simulink model "VCMGCM1962020b_v2"  (R2020b)
settings: Solver=FixedStepDiscrete  StartTime=0.0  StopTime=10.0  FixedStep=0.005  RelTol=1e-3  EnableMultiTasking=on
PreLoadFcn:
  | try, model_open; catch, disp('Error occurred while executing model pre-load callback: model_open.m'); disp('Please assure that the MATLAB working directory is set to the model directory before opening.'); end
InitFcn:
  | try, model_open; catch, end
undefined symbols (not defined in the file): Bridge, GCM, H, raptor_get_param_eval, raptor_get_safe_string, raptor_xcp_function
libraries: Blocks_lib x1165, Raptor_lib x665, simulink x62, VCM_lib x5
(part 7 of 23)

== system VCMGCM1962020b_v2/Fgnd/Virtual Sensors/Driver Inputs/Brk ==
  note: TBC
  Data : Inport
  BrkPos : Subsystem
  Bus Selector1 : BusSelector  OutputSignals=Sensors.Sensors.Driver.BrkSwInpt.BrkSwInptVld [Bool],Sensors.Sensors.Driver.BrkSwInpt.BrkSwInpt [Bool]
  Header : Blocks_lib/Header  width=Portrait  addtext=''
  Meas&Ovrd : Blocks_lib/Meas&Ovrd  nam='BrkSw'  name_source=Parameter  view_as=Number  enum_struct={}  gain=1  min=-inf  max=inf  precision=''  units='Bool'  help='Brake Switch position'  group='Virtual Sensors | Driver Input'
  Multiport Switch : MultiPortSwitch  DataPortOrder=Zero-based contiguous  Inputs=2  zeroidx=on
  Relational Operator : RelationalOperator  OutDataTypeStr=boolean  RndMeth=Simplest
  Zero-Order Hold : ZeroOrderHold  SampleTime=-1
  raptor_adjustment : Raptor_lib/Data Storage/raptor_adjustment  paramName='BrkSwSource'  nameSource=Parameter  initValue=0  dataType=double  storage=Calibration  calDispType=Number  calEnum={}  calGain=1.0  calOffset=0.0  calMax=inf  calMin=-inf  calFormat='-1'  calUnit='Bool'  calHelp=' 0 = simple switch., 1 = dual sensor switch'  calAccess=1  calFunction='Virtual Sensors | Driver Input'  calDispHeaders=off  calColHeaders={'Col1' 'Col2' 'Col3'}  calRowHeaders={'Row1' 'Row2' 'Row3'}
      settings: SourceProductName=Raptor
  raptor_adjustment1 : Raptor_lib/Data Storage/raptor_adjustment  paramName='BrkPos_Swtch_Thr'  nameSource=Parameter  initValue=20  dataType=double  storage=Calibration  calDispType=Number  calEnum={}  calGain=1.0  calOffset=0.0  calMax=inf  calMin=-inf  calFormat='-1'  calUnit='%'  calHelp=' Value of Pos Sensor to set Vitual brk switch to on'  calAccess=1  calFunction='Virtual Sensors | Driver Input'  calDispHeaders=off  calColHeaders={'Col1' 'Col2' 'Col3'}  calRowHeaders={'Row1' 'Row2' 'Row3'}
      settings: SourceProductName=Raptor
  Vld : Outport  VectorParamsAs1DForOutWhenUnconnected=off
  Brk : Outport  Port=2  VectorParamsAs1DForOutWhenUnconnected=off
  Pos : Outport  Port=3  VectorParamsAs1DForOutWhenUnconnected=off
  PosVld : Outport  Port=4  VectorParamsAs1DForOutWhenUnconnected=off
  wires:
  Data/1 -> BrkPos/1(Data), Bus Selector1/1
  Meas&Ovrd/1 -> Multiport Switch/2
  Bus Selector1/1 -> Zero-Order Hold/1  "<BrkSwInptVld [Bool]>"
  Bus Selector1/2 -> Meas&Ovrd/1  "<BrkSwInpt [Bool]>"
  Zero-Order Hold/1 -> Vld/1  "BrkSwVld [Bool]"
  BrkPos/1(Vld) -> PosVld/1
  BrkPos/2(%) -> Relational Operator/1, Pos/1
  raptor_adjustment1/1 -> Relational Operator/2
  raptor_adjustment/1 -> Multiport Switch/1
  Relational Operator/1 -> Multiport Switch/3
  Multiport Switch/1 -> Brk/1

== system VCMGCM1962020b_v2/Fgnd/Virtual Sensors/Driver Inputs/ParkBrake ==
  Data : Inport
  Bus Selector : BusSelector  OutputSignals=Sensors.CAN.Other.BCM.CCVS1_BCM.Parking_Brak_Switch.Parking_Brak_SwitchVld [Bool],Sensors.CAN.Other.BCM.CCVS1_BCM.Parking_Brak_Switch.Parking_Brak_Switch [enum]
  Constant : Constant
  Constant1 : Constant  Value=boolean(0)
  Constant2 : Constant  Value=boolean(1)
  Equal : RelationalOperator  Operator===  OutDataTypeStr=boolean  RndMeth=Simplest
  Header : Blocks_lib/Header  width=Portrait  addtext=''
  Multiport Switch : MultiPortSwitch  DataPortOrder=Zero-based contiguous  Inputs=2  zeroidx=on
  Multiport Switch1 : MultiPortSwitch  DataPortOrder=Zero-based contiguous  Inputs=2  zeroidx=on
  raptor_adjustment : Raptor_lib/Data Storage/raptor_adjustment  paramName='PrkBrk_Dflt'  nameSource=Parameter  initValue=0.00  dataType=boolean  storage=Calibration  calDispType=Number  calEnum={'False', 'True'}  calGain=1.0  calOffset=0.0  calMax=inf  calMin=-inf  calFormat='-1'  calUnit=''  calHelp=''  calAccess=1  calFunction=raptor_xcp_function(gcb)  calDispHeaders=off  calColHeaders={'Col1' 'Col2' 'Col3'}  calRowHeaders={'Row1' 'Row2' 'Row3'}
      settings: SourceProductName=Raptor
  raptor_measurement : Raptor_lib/Data Storage/raptor_measurement  paramName='PrkBrk'  nameSource=Parameter  calDispType=Number  calEnum={'False', 'True'}  calGain=1.0  calOffset=0.0  calMax=inf  calMin=-inf  calFormat='-1'  calUnit=''  calHelp=''  calAccess=1  calFunction=raptor_xcp_function(gcb)  calVisible=on
      settings: SourceProductName=Raptor
  Prk : Outport
  wires:
  Data/1 -> Bus Selector/1
  Bus Selector/2 -> Equal/1  "<Parking_Brak_Switch [enum]>"
  Constant/1 -> Equal/2
  Bus Selector/1 -> Multiport Switch/1  "<Parking_Brak_SwitchVld [Bool]>"
  Multiport Switch/1 -> Prk/1, raptor_measurement/1  "Prk [Bool]"
  Equal/1 -> Multiport Switch1/1
  Constant1/1 -> Multiport Switch1/2
  Constant2/1 -> Multiport Switch1/3
  Multiport Switch1/1 -> Multiport Switch/3
  raptor_adjustment/1 -> Multiport Switch/2

== system VCMGCM1962020b_v2/Fgnd/Virtual Sensors/Driver Inputs/VehPwrMode ==
  Data : Inport
  Bus Selector : BusSelector  OutputSignals=Sensors.Sensors.Volt.Wake [Bool]
  EnumCnst : Blocks_lib/EnumCnst  val='Off'  typ=uint8  enum=EnumLst.VehPwrMode
  EnumCnst1 : Blocks_lib/EnumCnst  val='Run'  typ=uint8  enum=EnumLst.VehPwrMode
  Header : Blocks_lib/Header  width=Portrait  addtext=''
  Multiport Switch : MultiPortSwitch  DataPortOrder=Zero-based contiguous  Inputs=2  zeroidx=on
  enum : Outport  VectorParamsAs1DForOutWhenUnconnected=off
  wires:
  Multiport Switch/1 -> enum/1
  Data/1 -> Bus Selector/1
  Bus Selector/1 -> Multiport Switch/1  "<Wake [Bool]>"
  EnumCnst/1 -> Multiport Switch/2
  EnumCnst1/1 -> Multiport Switch/3

== system VCMGCM1962020b_v2/Fgnd/Virtual Sensors/PDU/HVAccCur ==
  note: Note: This value is used downstream to calculate inverter and charger current limits.
      | Therefore, neither inverter nor charger current should be included in this calculation.
  Data : Inport
  Bus Selector : BusSelector  OutputSignals=VirtualSensors.DCDC.DCDCInptCur [A]
  Header : Blocks_lib/Header  width=Portrait  addtext=''
  raptor_measurement : Raptor_lib/Data Storage/raptor_measurement  paramName='HVAccCur'  nameSource=Parameter  calDispType=Number  calEnum={'Disabled', 'Enabled'}  calGain=1  calOffset=0  calMax=inf  calMin=-inf  calFormat=''  calUnit='A'  calHelp='High-voltage accessory current'  calAccess=1  calFunction='Virtual Sensors | PDU'  calVisible=on
      settings: SourceProductName=Raptor
  A : Outport  VectorParamsAs1DForOutWhenUnconnected=off
  wires:
  Data/1 -> Bus Selector/1
  Bus Selector/1 -> raptor_measurement/1, A/1  "<DCDCInptCur [A]>"

== system VCMGCM1962020b_v2/Fgnd/Virtual Sensors/PDU/HVBusIso ==
  Data : Inport
  Bus Selector : BusSelector  OutputSignals=Sensors.CAN.Batt.HVES1_Status1.PSV_ISO_TEST_State.PSV_ISO_TEST_StateVld [Bool],Sensors.CAN.Batt.HVES1_Status1.PSV_ISO_TEST_State.PSV_ISO_TEST_State []
  Compare To Constant : simulink/Logic and Bit Operations/Compare To Constant  relop=>=  const=4  OutDataTypeStr=boolean
  Compare To Constant1 : simulink/Logic and Bit Operations/Compare To Constant  relop=<=  const=5  OutDataTypeStr=boolean
  Header : Blocks_lib/Header  width=Portrait  addtext=''
  OR : Logic  Operator=OR  AllPortsSameDT=off  OutDataTypeStr=boolean
  Zero-Order Hold : ZeroOrderHold  SampleTime=-1
  Zero-Order Hold1 : ZeroOrderHold  SampleTime=-1
  Vld : Outport  VectorParamsAs1DForOutWhenUnconnected=off
  "ISOTst " : Outport  Port=2  VectorParamsAs1DForOutWhenUnconnected=off
  ISOFailed : Outport  Port=3  VectorParamsAs1DForOutWhenUnconnected=off
  wires:
  Data/1 -> Bus Selector/1
  Bus Selector/2 -> Compare To Constant1/1, Compare To Constant/1, Zero-Order Hold1/1  "<PSV_ISO_TEST_State []>"
  Bus Selector/1 -> Zero-Order Hold/1  "<PSV_ISO_TEST_StateVld [Bool]>"
  Zero-Order Hold/1 -> Vld/1
  Zero-Order Hold1/1 -> "ISOTst "/1  "PSV_ISO_Test_State [uint8]"
  Compare To Constant/1 -> OR/1
  Compare To Constant1/1 -> OR/2
  OR/1 -> ISOFailed/1

== system VCMGCM1962020b_v2/Fgnd/Virtual Sensors/PDU/HVBusVolt ==
  note: TBC
  Data : Inport
  Bus Selector : BusSelector  OutputSignals=Sensors.CAN.DrvInvtr.EM3.EM3DCv.EM3_InverterDcV.EM3_InverterDcVVld [Bool],Sensors.CAN.DrvInvtr.EM3.EM3DCv.EM3_InverterDcV.EM3_InverterDcV [V]
  HV Bus Voltage : Subsystem  Commented=on  mask{nam='HVBusVolt', group='Virtual Sensors | PDU'}
      mask prompts: nam "Name"
      mask Display: disp(['High-Voltage Bus Voltage\n' nam]);
  Header : Blocks_lib/Header  width=Portrait  addtext=''
  Vld : Outport  VectorParamsAs1DForOutWhenUnconnected=off
  V : Outport  Port=2  VectorParamsAs1DForOutWhenUnconnected=off
  wires:
  Data/1 -> Bus Selector/1, HV Bus Voltage/1(Data)
  Bus Selector/1 -> Vld/1  "<EM3_InverterDcVVld [Bool]>"
  Bus Selector/2 -> V/1  "<EM3_InverterDcV [V]>"

== system VCMGCM1962020b_v2/Fgnd/Virtual Sensors/PDU/MainCntrClosed ==
  Data : Inport
  Bus Selector : BusSelector  OutputSignals=VirtualSensors.PDU.MainPosCntrClosedVld [Bool],VirtualSensors.PDU.MainNegCntrClosedVld [Bool],VirtualSensors.PDU.MainPosCntrClosed [Bool],VirtualSensors.PDU.MainNegCntrClosed [Bool]
  Header : Blocks_lib/Header  width=Portrait  addtext=''
  Logical Operator : Logic  OutDataTypeStr=boolean
  Logical Operator1 : Logic  OutDataTypeStr=boolean
  Vld : Outport  VectorParamsAs1DForOutWhenUnconnected=off
  Bool : Outport  Port=2  VectorParamsAs1DForOutWhenUnconnected=off
  wires:
  Data/1 -> Bus Selector/1
  Bus Selector/1 -> Logical Operator/1  "<MainPosCntrClosedVld [Bool]>"
  Logical Operator/1 -> Vld/1
  Bus Selector/2 -> Logical Operator/2  "<MainNegCntrClosedVld [Bool]>"
  Bus Selector/3 -> Logical Operator1/1  "<MainPosCntrClosed [Bool]>"
  Bus Selector/4 -> Logical Operator1/2  "<MainNegCntrClosed [Bool]>"
  Logical Operator1/1 -> Bool/1

== system VCMGCM1962020b_v2/Fgnd/Virtual Sensors/Vehicle/Range ==
  Odom : Inport
  Data : Inport  Port=2
  Bus Selector : BusSelector  OutputSignals=VirtualSensors.Batt.BattSOC [%]
  CntrLoop : Subsystem  TreatAsAtomicUnit=on  mask(CntrLoop){init=0, typ=uint16, rstval=2000}
      mask prompts: init "Initial Value"; typ "Data Type"; rstval "Reset at:"
      mask init:
      | cb = gcb;
      | 
      | % --- Parameter Setting
      | set_param([cb '/Constant'], 'OutDataTypeStr', typ);
      mask TypeOptions typ: double | single | int8 | uint8 | int16 | uint16 | int32 | uint32 | boolean
      mask Display: disp(['Loop Counter\nReset at ' num2str(rstval)]);
  Compare To Constant : simulink/Logic and Bit Operations/Compare To Constant  relop===  const=0  OutDataTypeStr=boolean
  Filt : Blocks_lib/Filt  nam='RangeEstFiltTC'  group='Virtual Sensors | Speed'  samptime=samptime
  Header : Blocks_lib/Header  width=Portrait  addtext=''
  Product : Product
  RangeGain : Subsystem
  Subsystem1 : Subsystem
  raptor_measurement : Raptor_lib/Data Storage/raptor_measurement  paramName='VehRangeEst'  nameSource=Parameter  calDispType=Number  calEnum=EnumLst.VehDir  calGain=1  calOffset=0  calMax=inf  calMin=-inf  calFormat=''  calUnit='km'  calHelp='Estimated range to recharge required'  calAccess=1  calFunction='Virtual Sensors | Speed '  calVisible=on
      settings: SourceProductName=Raptor
  raptor_measurement1 : Raptor_lib/Data Storage/raptor_measurement  paramName='VehRangeParam'  nameSource=Parameter  calDispType=Number  calEnum=EnumLst.VehDir  calGain=1  calOffset=0  calMax=inf  calMin=-inf  calFormat=''  calUnit='km'  calHelp='Estimated range gain pre avg'  calAccess=1  calFunction='Virtual Sensors | Speed '  calVisible=on
      settings: SourceProductName=Raptor
  Range : Outport  VectorParamsAs1DForOutWhenUnconnected=off
  wires:
  Data/1 -> Bus Selector/1, RangeGain/2(data)
  Product/1 -> Filt/1
  Odom/1 -> RangeGain/1(Odom)
  RangeGain/1(DOdomDSoc) -> raptor_measurement1/1
  RangeGain/2(MvAv) -> Product/1
  Bus Selector/1 -> Product/2  "<BattSOC [%]>"
  Subsystem1/1(Rst) -> RangeGain/3(Rst)
  Subsystem1/2(Init) -> RangeGain/4(Init)
  CntrLoop/1(Count) -> Compare To Constant/1
  Compare To Constant/1 -> RangeGain/Enable
  Filt/1 -> Range/1, raptor_measurement/1

== system VCMGCM1962020b_v2/Fgnd/Virtual Sensors/Vehicle/VehDir ==
  Data : Inport
  Bus Selector : BusSelector  OutputSignals=VirtualSensors.DrvInvtr.DrvMtrSpd [rpm]
  Header : Blocks_lib/Header  width=Portrait  addtext=''
  Logical Operator : Logic  Operator=XOR  AllPortsSameDT=off  OutDataTypeStr=boolean
  RelOp(w/Hyst) : Blocks_lib/RelOp(w//Hyst)  relop=<=
  raptor_adjustment : Raptor_lib/Data Storage/raptor_adjustment  paramName='VehDirPolarity'  nameSource=Parameter  initValue=0  dataType=boolean  storage=Calibration  calDispType=Number  calEnum={'Disabled', 'Enabled'}  calGain=1  calOffset=0  calMax=inf  calMin=-inf  calFormat=''  calUnit='Bool'  calHelp='Vehicle direction polarity (flip to change polarity)'  calAccess=1  calFunction='Virtual Sensors | Speed'  calDispHeaders=off  calColHeaders={'Col1' 'Col2' 'Col3'}  calRowHeaders={'Row1' 'Row2' 'Row3'}
      settings: SourceProductName=Raptor
  raptor_adjustment1 : Raptor_lib/Data Storage/raptor_adjustment  paramName='VehDirThr'  nameSource=Parameter  initValue=[0 0]  dataType=double  storage=Calibration  calDispType=Number  calEnum={'Disabled', 'Enabled'}  calGain=1  calOffset=0  calMax=inf  calMin=-inf  calFormat=''  calUnit='rpm'  calHelp='Vehicle direction threshold'  calAccess=1  calFunction='Virtual Sensors | Speed'  calDispHeaders=off  calColHeaders={'Col1' 'Col2' 'Col3'}  calRowHeaders={'Row1' 'Row2' 'Row3'}
      settings: SourceProductName=Raptor
  raptor_measurement : Raptor_lib/Data Storage/raptor_measurement  paramName='VehDir'  nameSource=Parameter  calDispType=Enumeration  calEnum=EnumLst.VehDir  calGain=1  calOffset=0  calMax=inf  calMin=-inf  calFormat=''  calUnit='enum'  calHelp='Vehicle direction'  calAccess=1  calFunction='Virtual Sensors | Speed'  calVisible=on
      settings: SourceProductName=Raptor
  enum : Outport  VectorParamsAs1DForOutWhenUnconnected=off
  wires:
  Data/1 -> Bus Selector/1
  Logical Operator/1 -> raptor_measurement/1, enum/1
  Bus Selector/1 -> RelOp(w/Hyst)/1  "<DrvMtrSpd [rpm]>"
  raptor_adjustment1/1 -> RelOp(w/Hyst)/2
  raptor_adjustment/1 -> Logical Operator/2
  RelOp(w/Hyst)/1 -> Logical Operator/1

== system VCMGCM1962020b_v2/Fgnd/Virtual Sensors/Vehicle/VehOdmtr ==
  Data : Inport
  Add : Sum  InputSameDT=on  OutDataTypeStr=Inherit: Same as first input
  Bus Selector : BusSelector  OutputSignals=VirtualSensors.Spd.VehSpd [kph]
  Bus Selector1 : BusSelector  OutputSignals=Sensors.CAN.Other.Display.DisplayTG1.Trip_Reset.Trip_Reset [enum]
  Constant : Constant  Value=boolean(1)
  Gain : Gain  Gain=samptime / 3600
  Header : Blocks_lib/Header  width=Portrait  addtext=''
  RunSum : Blocks_lib/RunSum  nam='VehSpdSum'  storage=NonVolatile (EEPROM)  max=1000000
  Subsystem : Subsystem
  raptor_adjustment : Raptor_lib/Data Storage/raptor_adjustment  paramName='VehOdmtrInitVal'  nameSource=Parameter  initValue=0  dataType=double  storage=Calibration  calDispType=Number  calEnum={}  calGain=1  calOffset=0  calMax=inf  calMin=-inf  calFormat=''  calUnit='km'  calHelp='Vehicle odometer initial value'  calAccess=1  calFunction='Virtual Sensors | Speed'  calDispHeaders=off  calColHeaders={'Col1' 'Col2' 'Col3'}  calRowHeaders={'Row1' 'Row2' 'Row3'}
      settings: SourceProductName=Raptor
  raptor_measurement : Raptor_lib/Data Storage/raptor_measurement  paramName='VehOdmtrSpd'  nameSource=Parameter  calDispType=Number  calEnum={'Disabled', 'Enabled'}  calGain=1  calOffset=0  calMax=inf  calMin=-inf  calFormat=''  calUnit='km'  calHelp='Vehicle odometer (calculated by speed integration)'  calAccess=1  calFunction='Virtual Sensors | Speed'  calVisible=on
      settings: SourceProductName=Raptor
  raptor_measurement1 : Raptor_lib/Data Storage/raptor_measurement  paramName='VehOdmtr'  nameSource=Parameter  calDispType=Number  calEnum={'Disabled', 'Enabled'}  calGain=1  calOffset=0  calMax=inf  calMin=-inf  calFormat=''  calUnit='km'  calHelp='Vehicle odometer'  calAccess=1  calFunction='Virtual Sensors | Speed'  calVisible=on
      settings: SourceProductName=Raptor
  Trip : Outport  VectorParamsAs1DForOutWhenUnconnected=off
  km : Outport  Port=2  VectorParamsAs1DForOutWhenUnconnected=off
  wires:
  Gain/1 -> Add/1, raptor_measurement/1
  RunSum/1 -> Gain/1
  Constant/1 -> RunSum/1
  Add/1 -> Subsystem/1(Odom), raptor_measurement1/1, km/1
  raptor_adjustment/1 -> Add/2
  Data/1 -> Bus Selector1/1, Bus Selector/1
  Bus Selector/1 -> RunSum/2  "<VehSpd [kph]>"
  Bus Selector1/1 -> Subsystem/2(<Trip_Reset [enum]>)  "<Trip_Reset [enum]>"
  Subsystem/1(Trip) -> Trip/1

== system VCMGCM1962020b_v2/Fgnd/Virtual Sensors/Vehicle/VehSpd ==
  note: Note: if available, use speed reported from vehicle (eg, wheel speed-based from ABS module) as the primary value,
      | as this is a truer value and typically more stable than the motor speed-based value.
  Data : Inport
  Arb : Blocks_lib/Arb  nam='VehSpd'  units='kph'  eqn='u(1)'  minmax=min  samptime=samptime
  Header : Blocks_lib/Header  width=Portrait  addtext=''
  Motor Speed-Based : Subsystem
  WSS Based : Subsystem
  raptor_measurement : Raptor_lib/Data Storage/raptor_measurement  paramName='VehSpd'  nameSource=Parameter  calDispType=Number  calEnum={'Disabled', 'Enabled'}  calGain=1  calOffset=0  calMax=inf  calMin=-inf  calFormat=''  calUnit='kph'  calHelp='Vehicle speed'  calAccess=1  calFunction='Virtual Sensors | Speed'  calVisible=on
      settings: SourceProductName=Raptor
  Vld : Outport  VectorParamsAs1DForOutWhenUnconnected=off
  kph : Outport  Port=2  VectorParamsAs1DForOutWhenUnconnected=off
  wires:
  Data/1 -> WSS Based/1(In1), Motor Speed-Based/1(Data)
  Arb/1 -> Vld/1
  Arb/2 -> raptor_measurement/1, kph/1
  WSS Based/1(Vld) -> Arb/1
  Motor Speed-Based/2(Spd [kph]) -> Arb/4
  Motor Speed-Based/1(Vld) -> Arb/2
  WSS Based/2(Spd [kph]) -> Arb/3

== system VCMGCM1962020b_v2/Fgnd/Actuators/Actuators/Other/Cmd Inversion ==
  <CoolPump1SpdReq [%]> : Inport
  raptor_table_1d : Raptor_lib/Table Lookup/raptor_table_1d  dataName='PumpCmdInversion'  initValue=[ 95 5]  dataType=double  storage=Calibration  initValueX=[ 5 95]  dataTypeXY=double  storageXY=Calibration  calVisible=on  showTable=on  calGain=1.0  calOffset=0.0  calMax=Inf  calMin=-Inf  calFormat='-1'  calUnit='%'  calHelp='Invertes teh pump DC command since LS driver'  showBreakpoint=on  dataNameX='PumpCmdInversionX'  calGainX=1  calOffsetX=0.0  calMaxX=Inf  calMinX=-Inf  calFormatX='-1'  calUnitX=''  calHelpX=''  calAccess=1  calFunction="'Actuators  | Pumps'"  measureEnable=off  mName=[raptor_get_param_eval(gcb,'dataName'), '_Output']
      settings: SourceProductName=Raptor
  Out1 : Outport
  wires:
  raptor_table_1d/1 -> Out1/1
  <CoolPump1SpdReq [%]>/1 -> raptor_table_1d/1

== system VCMGCM1962020b_v2/Fgnd/Actuators/CAN/Battery/ChgrBatt_State_Transition_Cmd ==
  Data : Inport
  Bus Selector : BusSelector  OutputSignals=Control.Mode.StartStop.CANDiagEnbl [Bool]
  CANTxMsgEnbl : Blocks_lib/CANTxMsgEnbl  custom=on  custom_nam=[nam '---']  msgnam=ChgrBatt_State_Transition_Cmd
  Header : Blocks_lib/Header  width=Portrait  addtext=''
  MsgTx : Subsystem
  wires:
  Bus Selector/1 -> CANTxMsgEnbl/1  "<CANDiagEnbl [Bool]>"
  CANTxMsgEnbl/1 -> MsgTx/Enable
  Data/1 -> Bus Selector/1, MsgTx/1(Data)

== system VCMGCM1962020b_v2/Fgnd/Actuators/CAN/Battery/MsgName ==
  Data : Inport
  Bus Selector : BusSelector  OutputSignals=Control.Mode.StartStop.CANDiagEnbl [Bool]
  CANTxMsgEnbl : Blocks_lib/CANTxMsgEnbl  custom=on  custom_nam=[nam '---']  msgnam=ChgrBCH1
  Header : Blocks_lib/Header  width=Portrait  addtext=''
  MsgTx : Subsystem
  wires:
  Bus Selector/1 -> CANTxMsgEnbl/1  "<CANDiagEnbl [Bool]>"
  CANTxMsgEnbl/1 -> MsgTx/Enable
  Data/1 -> Bus Selector/1, MsgTx/1(Data)

== system VCMGCM1962020b_v2/Fgnd/Actuators/CAN/Body Control/BCMBCH1 ==
  Data : Inport
  Bus Selector : BusSelector  OutputSignals=Control.Mode.StartStop.ModWake [Bool]
  CANTxMsgEnbl : Blocks_lib/CANTxMsgEnbl  custom=on  custom_nam=[nam '---']  msgnam=BCMBCH1
  Header : Blocks_lib/Header  width=Portrait  addtext=''
  MsgTx : Subsystem
  wires:
  Bus Selector/1 -> CANTxMsgEnbl/1  "<ModWake [Bool]>"
  CANTxMsgEnbl/1 -> MsgTx/Enable
  Data/1 -> Bus Selector/1, MsgTx/1(Data)

== system VCMGCM1962020b_v2/Fgnd/Actuators/CAN/Body Control/BCMCCVS1_VCU ==
  Data : Inport
  Bus Selector : BusSelector  OutputSignals=Control.Mode.StartStop.ModWake [Bool]
  CANTxMsgEnbl : Blocks_lib/CANTxMsgEnbl  custom=on  custom_nam=[nam '---']  msgnam=BCMCCVS1_VCU
  Header : Blocks_lib/Header  width=Portrait  addtext=''
  MsgTx : Subsystem
  wires:
  Bus Selector/1 -> CANTxMsgEnbl/1  "<ModWake [Bool]>"
  CANTxMsgEnbl/1 -> MsgTx/Enable
  Data/1 -> Bus Selector/1, MsgTx/1(Data)

== system VCMGCM1962020b_v2/Fgnd/Actuators/CAN/Body Control/BCMCM3 ==
  Data : Inport
  Bus Selector : BusSelector  OutputSignals=Control.Mode.StartStop.ModWake [Bool]
  CANTxMsgEnbl : Blocks_lib/CANTxMsgEnbl  custom=on  custom_nam=[nam '---']  msgnam=BCMCM3
  Header : Blocks_lib/Header  width=Portrait  addtext=''
  MsgTx : Subsystem
  wires:
  Bus Selector/1 -> CANTxMsgEnbl/1  "<ModWake [Bool]>"
  CANTxMsgEnbl/1 -> MsgTx/Enable
  Data/1 -> Bus Selector/1

== system VCMGCM1962020b_v2/Fgnd/Actuators/CAN/Body Control/BCMETC2 ==
  Data : Inport
  Bus Selector : BusSelector  OutputSignals=Control.Mode.StartStop.ModWake [Bool]
  CANTxMsgEnbl : Blocks_lib/CANTxMsgEnbl  custom=on  custom_nam=[nam '---']  msgnam=BCMETC2
  Header : Blocks_lib/Header  width=Portrait  addtext=''
  MsgTx : Subsystem
  wires:
  Bus Selector/1 -> CANTxMsgEnbl/1  "<ModWake [Bool]>"
  CANTxMsgEnbl/1 -> MsgTx/Enable
  Data/1 -> Bus Selector/1, MsgTx/1(Data)

== system VCMGCM1962020b_v2/Fgnd/Actuators/CAN/Body Control/BCMICMSTS ==
  Data : Inport
  Bus Selector : BusSelector  OutputSignals=Control.Mode.StartStop.ModWake [Bool]
  CANTxMsgEnbl : Blocks_lib/CANTxMsgEnbl  custom=on  custom_nam=[nam '---']  msgnam=BCMICMSTS
  Header : Blocks_lib/Header  width=Portrait  addtext=''
  MsgTx : Subsystem
  wires:
  Bus Selector/1 -> CANTxMsgEnbl/1  "<ModWake [Bool]>"
  CANTxMsgEnbl/1 -> MsgTx/Enable
  Data/1 -> Bus Selector/1, MsgTx/1(Data)

== system VCMGCM1962020b_v2/Fgnd/Actuators/CAN/Body Control/BCMVEP2 ==
  Data : Inport
  Bus Selector : BusSelector  OutputSignals=Control.Mode.StartStop.ModWake [Bool]
  CANTxMsgEnbl : Blocks_lib/CANTxMsgEnbl  custom=on  custom_nam=[nam '---']  msgnam=BCMVEP2
  Header : Blocks_lib/Header  width=Portrait  addtext=''
  MsgTx : Subsystem
  wires:
  Bus Selector/1 -> CANTxMsgEnbl/1  "<ModWake [Bool]>"
  CANTxMsgEnbl/1 -> MsgTx/Enable
  Data/1 -> Bus Selector/1, MsgTx/1(Data)

== system VCMGCM1962020b_v2/Fgnd/Actuators/CAN/Body Control/MsgName ==
  Data : Inport
  Bus Selector : BusSelector  OutputSignals=Control.Mode.StartStop.ModWake [Bool]
  CANTxMsgEnbl : Blocks_lib/CANTxMsgEnbl  custom=on  custom_nam=[nam '---']  msgnam=BCMICMSTS
  Header : Blocks_lib/Header  width=Portrait  addtext=''
  MsgTx : Subsystem
  wires:
  Bus Selector/1 -> CANTxMsgEnbl/1  "<ModWake [Bool]>"
  CANTxMsgEnbl/1 -> MsgTx/Enable
  Data/1 -> Bus Selector/1, MsgTx/1(Data)

== system VCMGCM1962020b_v2/Fgnd/Actuators/CAN/CCS Interface/CCSEV_ChargeParameters1 ==
  Data : Inport
  Bus Selector : BusSelector  OutputSignals=Control.Mode.StartStop.ChgCycle [Bool],Control.Mode.StartStop.ModWake [Bool]
  CANTxMsgEnbl : Blocks_lib/CANTxMsgEnbl  custom=on  custom_nam=[nam '---']  msgnam=CCSEV_ChargeParameters1
  Header : Blocks_lib/Header  width=Portrait  addtext=''
  Logical Operator : Logic  AllPortsSameDT=off  OutDataTypeStr=boolean
  MsgTx : Subsystem
  wires:
  Data/1 -> Bus Selector/1, MsgTx/1(Data)
  CANTxMsgEnbl/1 -> MsgTx/Enable
  Bus Selector/1 -> Logical Operator/1  "<ChgCycle [Bool]>"
  Bus Selector/2 -> Logical Operator/2  "<ModWake [Bool]>"
  Logical Operator/1 -> CANTxMsgEnbl/1

== system VCMGCM1962020b_v2/Fgnd/Actuators/CAN/CCS Interface/CCSEV_ChargeParameters2 ==
  Data : Inport
  Bus Selector : BusSelector  OutputSignals=Control.Mode.StartStop.ChgCycle [Bool],Control.Mode.StartStop.ModWake [Bool]
  CANTxMsgEnbl : Blocks_lib/CANTxMsgEnbl  custom=on  custom_nam=[nam '---']  msgnam=CCSEV_ChargeParameters2
  Header : Blocks_lib/Header  width=Portrait  addtext=''
  Logical Operator : Logic  AllPortsSameDT=off  OutDataTypeStr=boolean
  MsgTx : Subsystem
  wires:
  CANTxMsgEnbl/1 -> MsgTx/Enable
  Data/1 -> Bus Selector/1, MsgTx/1(Data)
  Bus Selector/1 -> Logical Operator/1  "<ChgCycle [Bool]>"
  Bus Selector/2 -> Logical Operator/2  "<ModWake [Bool]>"
  Logical Operator/1 -> CANTxMsgEnbl/1

== system VCMGCM1962020b_v2/Fgnd/Actuators/CAN/CCS Interface/CCSEV_DC_ChargeInfo1 ==
  Data : Inport
  Cmd : Inport  Port=2
  Bus Selector : BusSelector  OutputSignals=Control.Mode.StartStop.ChgCycle [Bool],Control.Mode.StartStop.ModWake [Bool]
  CANTxMsgEnbl : Blocks_lib/CANTxMsgEnbl  custom=on  custom_nam=[nam '---']  msgnam=CCSEV_DC_ChargeInfo1
  Header : Blocks_lib/Header  width=Portrait  addtext=''
  Logical Operator : Logic  AllPortsSameDT=off  OutDataTypeStr=boolean
  MsgTx : Subsystem
  wires:
  CANTxMsgEnbl/1 -> MsgTx/Enable
  Data/1 -> Bus Selector/1, MsgTx/1(Data)
  Cmd/1 -> MsgTx/2(Cmd)
  Bus Selector/1 -> Logical Operator/1  "<ChgCycle [Bool]>"
  Bus Selector/2 -> Logical Operator/2  "<ModWake [Bool]>"
  Logical Operator/1 -> CANTxMsgEnbl/1

== system VCMGCM1962020b_v2/Fgnd/Actuators/CAN/CCS Interface/Commands ==
  Data : Inport
  Bus Creator : BusCreator  Inputs=7
  Bus Selector : BusSelector  OutputSignals=Control.Mode.StartStop.ChgMode [Bool],Sensors.CAN.CCS.CCSM2IEV_Command.CCSCurrentState.CCSCurrentState [Enum],VirtualSensors.PDU.HVBusVolt [V],Control.Chgr.ChgrDCVoltSetpt [V],Control.Chgr.OffBoardChgrDCCurLim [A],Sensors.CAN.CCS.CCSM2IEV_Command.CCSDC_CloseContactorsRequest.CCSDC_CloseContactorsRequest [Boolean]
  Charge Port DC Voltage Diag : Subsystem
  Charge Port DC Voltage/Current : Subsystem
  Commands : Stateflow chart  TreatAsAtomicUnit=on
  DC Charge Contactors : Subsystem
  Header : Blocks_lib/Header  width=Portrait  addtext=''
  raptor_adjustment : Raptor_lib/Data Storage/raptor_adjustment  paramName='EVTargetCurrentPreChg'  nameSource=Parameter  initValue=0  dataType=double  storage=Calibration  calDispType=Number  calEnum={'False', 'True'}  calGain=1.0  calOffset=0.0  calMax=inf  calMin=-inf  calFormat='-1'  calUnit='A'  calHelp='EV target current (during EVSE pre-charge)'  calAccess=1  calFunction=['Actuators | CAN | ' nam]  calDispHeaders=off  calColHeaders={'Col1' 'Col2' 'Col3'}  calRowHeaders={'Row1' 'Row2' 'Row3'}
      settings: SourceProductName=Raptor
  raptor_adjustment1 : Raptor_lib/Data Storage/raptor_adjustment  paramName='BattIsoTestDsblTime'  nameSource=Parameter  initValue=0  dataType=double  storage=Calibration  calDispType=Number  calEnum={'Disabled', 'Enabled'}  calGain=samptime  calOffset=0  calMax=inf  calMin=-inf  calFormat='0.3'  calUnit='sec'  calHelp='Battery isolation test disable time'  calAccess=1  calFunction=['Actuators | CAN | ' nam]  calDispHeaders=off  calColHeaders={'Col1' 'Col2' 'Col3'}  calRowHeaders={'Row1' 'Row2' 'Row3'}
      settings: SourceProductName=Raptor
  raptor_adjustment2 : Raptor_lib/Data Storage/raptor_adjustment  paramName='EVTargetCurrentRampInRate'  nameSource=Parameter  initValue=0 * samptime  dataType=double  storage=Calibration  calDispType=Number  calEnum={'Disabled', 'Enabled'}  calGain=1/samptime  calOffset=0  calMax=inf  calMin=-inf  calFormat=''  calUnit='A/s'  calHelp='EV target current ramp in rate'  calAccess=1  calFunction=['Actuators | CAN | ' nam]  calDispHeaders=off  calColHeaders={'Col1' 'Col2' 'Col3'}  calRowHeaders={'Row1' 'Row2' 'Row3'}
      settings: SourceProductName=Raptor
  raptor_adjustment3 : Raptor_lib/Data Storage/raptor_adjustment  paramName='EVTargetCurrentRampOutRate'  nameSource=Parameter  initValue=0 * samptime  dataType=double  storage=Calibration  calDispType=Number  calEnum={'Disabled', 'Enabled'}  calGain=1/samptime  calOffset=0  calMax=inf  calMin=-inf  calFormat=''  calUnit='A/s'  calHelp='EV target current ramp out rate'  calAccess=1  calFunction=['Actuators | CAN | ' nam]  calDispHeaders=off  calColHeaders={'Col1' 'Col2' 'Col3'}  calRowHeaders={'Row1' 'Row2' 'Row3'}
      settings: SourceProductName=Raptor
  raptor_adjustment4 : Raptor_lib/Data Storage/raptor_adjustment  paramName='ChgPortDCCurZeroMxTime'  nameSource=Parameter  initValue=0  dataType=double  storage=Calibration  calDispType=Number  calEnum={'Disabled', 'Enabled'}  calGain=samptime  calOffset=0  calMax=inf  calMin=-inf  calFormat='0.3'  calUnit='sec'  calHelp='Charge port DC current zero maximum time'  calAccess=1  calFunction=['Actuators | CAN | ' nam]  calDispHeaders=off  calColHeaders={'Col1' 'Col2' 'Col3'}  calRowHeaders={'Row1' 'Row2' 'Row3'}
      settings: SourceProductName=Raptor
  raptor_measurement : Raptor_lib/Data Storage/raptor_measurement  paramName='CCSCommandsStep'  nameSource=Parameter  calDispType=Number  calEnum={}  calGain=1.0  calOffset=0.0  calMax=inf  calMin=-inf  calFormat='-1'  calUnit=''  calHelp='CCS commands step'  calAccess=1  calFunction=['Actuators | CAN | ' nam]  calVisible=on
      settings: SourceProductName=Raptor
  Cmds : Outport  VectorParamsAs1DForOutWhenUnconnected=off
  wires:
  Charge Port DC Voltage/Current/3(CurZero) -> Commands/9(ChgPortDCCurZero)
  Commands/5(BattIsoTestDsbl) -> Bus Creator/5  "BattIsoTestDsbl [Bool]"
  raptor_adjustment1/1 -> Commands/13(BattIsoTestDsblTime)
  Commands/8(ChgPortDCVoltHiDiagEnbl) -> Charge Port DC Voltage Diag/1(DiagEnbl)
  raptor_adjustment4/1 -> Commands/16(ChgPortDCCurZeroMxTime)
  DC Charge Contactors/2(Open) -> Commands/11(DCChgCntrOpen)
  DC Charge Contactors/1(Closed) -> Commands/10(DCChgCntrClosed)
  Data/1 -> Charge Port DC Voltage/Current/1(Data), DC Charge Contactors/1(Data), Charge Port DC Voltage Diag/2(Data), Bus Selector/1
  Bus Selector/6 -> Commands/6(DC_CloseContactorsRequest)  "<CCSDC_CloseContactorsRequest [Boolean]>"
  Bus Selector/5 -> Commands/5(ChgrDCCurLim)  "<OffBoardChgrDCCurLim [A]>"
  Bus Selector/4 -> Commands/4(ChgrDCVoltSetpt)  "<ChgrDCVoltSetpt [V]>"
  Bus Selector/3 -> Commands/3(HVBusVolt)  "<HVBusVolt [V]>"
  Bus Selector/1 -> Commands/1(ChgMode)  "<ChgMode [Bool]>"
  Bus Selector/2 -> Commands/2(CurrentState)  "<CCSCurrentState [Enum]>"
  Charge Port DC Voltage/Current/2(VoltZero) -> Commands/8(ChgPortDCVoltZero)
  Charge Port DC Voltage/Current/1(VoltMatch) -> Commands/7(ChgPortDCVoltMatch)
  raptor_adjustment3/1 -> Commands/15(EVTargetCurrentRampOutRate)
  raptor_adjustment2/1 -> Commands/14(EVTargetCurrentRampInRate)
  raptor_adjustment/1 -> Commands/12(EVTargetCurrentPreChg)
  Bus Creator/1 -> Cmds/1  "Cmd"
  Commands/7(DC_ContactorsState) -> Bus Creator/7  "DC_ContactorsState [Bool]"
  Commands/6(DCChgCntr) -> Bus Creator/6  "DCChgCntr [Bool]"
  Commands/4(EVTargetCurrent) -> Bus Creator/4  "EVTargetCurrent [A]"
  Commands/3(EVTargetVoltage) -> Bus Creator/3  "EVTargetVoltage [V]"
  Commands/2(Command) -> Bus Creator/2  "Command [enum]"
  Commands/1(Step) -> Bus Creator/1, raptor_measurement/1  "CommandsStep [enum]"

== system VCMGCM1962020b_v2/Fgnd/Actuators/CAN/CCS Interface/MsgName ==
  Data : Inport
  Cmd : Inport  Port=2
  Bus Selector : BusSelector  OutputSignals=Control.Mode.StartStop.ChgCycle [Bool],Control.Mode.StartStop.ModWake [Bool]
  CANTxMsgEnbl : Blocks_lib/CANTxMsgEnbl  custom=on  custom_nam=[nam '---']  msgnam=CCSBCC_Command
  Header : Blocks_lib/Header  width=Portrait  addtext=''
  Logical Operator : Logic  AllPortsSameDT=off  OutDataTypeStr=boolean
  MsgTx : Subsystem
  SleepMsgTx : Subsystem
  wires:
  Data/1 -> Bus Selector/1
  Cmd/1 -> MsgTx/1(Cmd)
  CANTxMsgEnbl/1 -> SleepMsgTx/Trigger, MsgTx/Enable
  Bus Selector/1 -> Logical Operator/1  "<ChgCycle [Bool]>"
  Bus Selector/2 -> Logical Operator/2  "<ModWake [Bool]>"
  Logical Operator/1 -> CANTxMsgEnbl/1

== system VCMGCM1962020b_v2/Fgnd/Actuators/CAN/Charger/ChgrBMSA ==
  Data : Inport
  Bus Selector : BusSelector  OutputSignals=Control.Mode.StartStop.ChgCycle [Bool]
  CANTxMsgEnbl : Blocks_lib/CANTxMsgEnbl  custom=on  custom_nam=[nam '---']  msgnam=ChgrBMSA
  Header : Blocks_lib/Header  width=Portrait  addtext=''
  MsgTx : Subsystem
  wires:
  Bus Selector/1 -> CANTxMsgEnbl/1  "<ChgCycle [Bool]>"
  CANTxMsgEnbl/1 -> MsgTx/Enable
  Data/1 -> Bus Selector/1, MsgTx/1(Data)

== system VCMGCM1962020b_v2/Fgnd/Actuators/CAN/Charger/Config Msgs ==
  Config Sequence : Subsystem
  Header : Blocks_lib/Header  width=Portrait  addtext=''
  raptor_adjustment : Raptor_lib/Data Storage/raptor_adjustment  paramName='ChgrConfigEnbl'  nameSource=Parameter  initValue=0  dataType=boolean  storage=Calibration  calDispType=Number  calEnum={'False', 'True'}  calGain=1  calOffset=0  calMax=inf  calMin=-inf  calFormat=''  calUnit='Bool'  calHelp='CAN message enable'  calAccess=1  calFunction='Actuators | Enables'  calDispHeaders=off  calColHeaders={'Col1' 'Col2' 'Col3'}  calRowHeaders={'Row1' 'Row2' 'Row3'}
      settings: SourceProductName=Raptor
  wires:
  raptor_adjustment/1 -> Config Sequence/Enable

== system VCMGCM1962020b_v2/Fgnd/Actuators/CAN/DC//DC Converter/MsgName ==
  Data : Inport
  Bus Selector : BusSelector  OutputSignals=Control.Other.Other.SysWake [Bool]
  CANTxMsgEnbl : Blocks_lib/CANTxMsgEnbl  custom=on  custom_nam=[nam '---']  msgnam=DCDCOutputSetpoint0
  Header : Blocks_lib/Header  width=Portrait  addtext=''
  MsgTx : Subsystem
  wires:
  CANTxMsgEnbl/1 -> MsgTx/Enable
  Bus Selector/1 -> CANTxMsgEnbl/1  "<SysWake [Bool]>"
  Data/1 -> Bus Selector/1, MsgTx/1(Data)

== system VCMGCM1962020b_v2/Fgnd/Actuators/CAN/DC//DC Converter1/DCDCDCDC_Cmmd_0_16V ==
  Data : Inport
  Bus Selector : BusSelector  OutputSignals=Control.Other.Other.SysWake [Bool]
  CANTxMsgEnbl : Blocks_lib/CANTxMsgEnbl  custom=on  custom_nam=[nam '---']  msgnam=DCDCDCDC_Cmmd_0_16V
  Header : Blocks_lib/Header  width=Portrait  addtext=''
  MsgTx : Subsystem
  wires:
  CANTxMsgEnbl/1 -> MsgTx/Enable
  Bus Selector/1 -> CANTxMsgEnbl/1  "<SysWake [Bool]>"
  Data/1 -> Bus Selector/1, MsgTx/1(Data)

== system VCMGCM1962020b_v2/Fgnd/Actuators/CAN/Display/DisplayHVES1_D2 ==
  Data : Inport
  Bus Selector : BusSelector  OutputSignals=Control.Other.Other.SysWake [Bool]
  CANTxMsgEnbl : Blocks_lib/CANTxMsgEnbl  custom=on  custom_nam=[nam '---']  msgnam=DisplayHVES1_D2
  Header : Blocks_lib/Header  width=Portrait  addtext=''
  MsgTx : Subsystem
  wires:
  CANTxMsgEnbl/1 -> MsgTx/Enable
  Bus Selector/1 -> CANTxMsgEnbl/1  "<SysWake [Bool]>"
  Data/1 -> Bus Selector/1, MsgTx/1(Data)

== system VCMGCM1962020b_v2/Fgnd/Actuators/CAN/Drive Inverter/DrvInvtrNMT ==
  State : Inport
  Data : Inport  Port=2
  Bus Selector : BusSelector  OutputSignals=Control.Other.Other.SysWake [Bool]
  Bus Selector1 : BusSelector  OutputSignals=NMTXmit
  CANTxMsgEnbl : Blocks_lib/CANTxMsgEnbl  custom=on  custom_nam=[nam '---']  msgnam=DrvInvtrNMT
  Header : Blocks_lib/Header  width=Portrait  addtext=''
  Logical Operator : Logic  AllPortsSameDT=off  OutDataTypeStr=boolean
  MsgTx : Subsystem
  OR : Logic  Operator=OR  AllPortsSameDT=off  OutDataTypeStr=boolean
  wires:
  CANTxMsgEnbl/1 -> MsgTx/Trigger
  Data/1 -> Bus Selector/1
  Bus Selector1/1 -> Logical Operator/2  "<NMTXmit>"
  State/1 -> MsgTx/1(State), Bus Selector1/1
  [Bypass_Sys_Wake] -> OR/1
  Bus Selector/1 -> Logical Operator/1  "<SysWake [Bool]>"
  Logical Operator/1 -> OR/2
  OR/1 -> CANTxMsgEnbl/1

== system VCMGCM1962020b_v2/Fgnd/Actuators/CAN/Drive Inverter/DrvInvtrVCU1 ==
  State : Inport
  Data : Inport  Port=2
  Bus Selector : BusSelector  OutputSignals=Control.Other.Other.SysWake [Bool]
  CANTxMsgEnbl : Blocks_lib/CANTxMsgEnbl  custom=on  custom_nam=[nam '---']  msgnam=DrvInvtrVCU1
  Header : Blocks_lib/Header  width=Portrait  addtext=''
  Logical Operator1 : Logic  Operator=OR  AllPortsSameDT=off  OutDataTypeStr=boolean
  MsgTx : Subsystem
  raptor_adjustment2 : Raptor_lib/Data Storage/raptor_adjustment  paramName='BypassSystemWake_IntestMode'  nameSource=Parameter  initValue=1  dataType=boolean  storage=Calibration  calDispType=Number  calEnum={'False', 'True'}  calGain=samptime  calOffset=0.0  calMax=inf  calMin=-inf  calFormat='-1'  calUnit='sec'  calHelp='Set to 1 to turn on subsystems befor system wake is active'  calAccess=1  calFunction=['Actuators | CAN | ' msgnam]  calDispHeaders=off  calColHeaders={'Col1' 'Col2' 'Col3'}  calRowHeaders={'Row1' 'Row2' 'Row3'}
      settings: SourceProductName=Raptor
  raptor_data_def : Raptor_lib/Data Storage/raptor_data_def  Commented=on  dataName='BypassSystemWake'  initValue=0  dataType=double  storage=Volatile (RAM)  calVisible=on  calType=Measurement  calDispType=Number  calEnum={'False', 'True'}  calGain=1.0  calOffset=0  calMin=-inf  calMax=inf  calFormat='-1'  calUnit=''  calHelp=''  calAccess=1  calFunction=raptor_xcp_function(gcb)  calDispHeaders=off  calColHeaders={'Col1' 'Col2' 'Col3'}  calRowHeaders={'Row1' 'Row2' 'Row3'}
      settings: SourceProductName=Raptor
  raptor_data_write : Raptor_lib/Data Storage/raptor_data_write  Commented=on  dataName='BypassSystemWake'  dataShape=Scalar  idxSource=Input Port  idxRow=1  idxCol=1
      settings: SourceProductName=Raptor
  tag scope: Bypass_Sys_Wake=global
  wires:
  CANTxMsgEnbl/1 -> MsgTx/Enable
  Bus Selector/1 -> Logical Operator1/2  "<SysWake [Bool]>"
  Logical Operator1/1 -> CANTxMsgEnbl/1
  Data/1 -> Bus Selector/1
  State/1 -> MsgTx/1(State)
  raptor_adjustment2/1 -> raptor_data_write/1, [Bypass_Sys_Wake], Logical Operator1/1

== system VCMGCM1962020b_v2/Fgnd/Actuators/CAN/Drive Inverter/DrvInvtrVCU2 ==
  State : Inport
  Data : Inport  Port=2
  Bus Selector : BusSelector  OutputSignals=Control.Other.Other.SysWake [Bool]
  CANTxMsgEnbl : Blocks_lib/CANTxMsgEnbl  custom=on  custom_nam=[nam '---']  msgnam=DrvInvtrVCU2
  Header : Blocks_lib/Header  width=Portrait  addtext=''
  MsgTx : Subsystem
  OR : Logic  Operator=OR  AllPortsSameDT=off  OutDataTypeStr=boolean
  wires:
  CANTxMsgEnbl/1 -> MsgTx/Enable
  Data/1 -> Bus Selector/1
  OR/1 -> CANTxMsgEnbl/1
  State/1 -> MsgTx/1(State)
  Bus Selector/1 -> OR/2  "<SysWake [Bool]>"
  [Bypass_Sys_Wake] -> OR/1

== system VCMGCM1962020b_v2/Fgnd/Actuators/CAN/Drive Inverter/Function-Call Subsystem ==
  function : TriggerPort  TriggerType=function-call  VariantControl=(inherit)
  MsgName : Subsystem
      mask help:
      | Example of how to set up a CAN message transmit.
      | 1. Copy this block into the main model.
      | 2. Disable/break library link.
      | 3. Underneath, set up CAN Tx Message block.
      | 4. For each field, connect a CANTxField block from the CAN block to the bus creator; adjust parameters as necessary.
      mask init:
      | [msgnam, msgbus] = CANBlockInit('Tx');
      mask Display: disp(['CAN Tx: Message\n' msgnam '\n' msgbus]);

== system VCMGCM1962020b_v2/Fgnd/Actuators/CAN/Drive Inverter/NMT Trasition Command ==
  note: TBC: THis needs to be updated per the Saietta interface
      | NOte: WE will use the simple Autostart feature of the drive inverter.
      | THis enables starting without the NMT message handshake
      |
      | Process:
      | Wake all modules
      | Close battery contactors
      | Reset inverter faults
      | Send VCU1/VCU2 Messages
      | Enable inverter in Torque mode.
  NMT_Step : Inport
  Data : Inport  Port=2
  Bus Creator1 : BusCreator  Inputs=7
  Bus Selector : BusSelector  OutputSignals=Control.DrvInvtr.MtrTrqReq.DrvInvtr.DrvMtrTrqReq [Nm]
  Bus Selector1 : BusSelector  OutputSignals=VCU1StateCmd [bool],TrqCmd [Nm],SpdCmd [rpm],VCU1_2_Transmit [bool],NMT_Xmit [bool],NMT_Target_Node,NMT_StateDmd
  Error : Subsystem  TreatAsAtomicUnit=on
  Error1 : Subsystem  TreatAsAtomicUnit=on
  Error2 : Subsystem  TreatAsAtomicUnit=on
  Header : Blocks_lib/Header  width=Portrait  addtext=''
  Init State : Subsystem  TreatAsAtomicUnit=on
  Inverter Error Reset : Subsystem
  Meas&Ovrd : Blocks_lib/Meas&Ovrd  nam=[nam 'AppStateCmd']  name_source=Parameter  view_as=Number  enum_struct={}  gain=1  min=-inf  max=inf  precision=''  units=''  help='CAN message value'  group=['Actuators | CAN | ' nam]
  Meas&Ovrd1 : Blocks_lib/Meas&Ovrd  nam=[nam 'StateTrqCmd']  name_source=Parameter  view_as=Number  enum_struct={}  gain=1  min=-inf  max=inf  precision=''  units=''  help='CAN message value'  group=['Actuators | CAN | ' nam]
  Meas&Ovrd2 : Blocks_lib/Meas&Ovrd  nam=[nam 'StateSpdCmd']  name_source=Parameter  view_as=Number  enum_struct={}  gain=1  min=-inf  max=inf  precision=''  units=''  help='CAN message value'  group=['Actuators | CAN | ' nam]
  Meas&Ovrd3 : Blocks_lib/Meas&Ovrd  nam=[nam 'VCU12Xmit']  name_source=Parameter  view_as=Number  enum_struct={}  gain=1  min=-inf  max=inf  precision=''  units=''  help='CAN message value'  group=['Actuators | CAN | ' nam]
  Meas&Ovrd4 : Blocks_lib/Meas&Ovrd  nam=[nam 'NMT_Xmit']  name_source=Parameter  view_as=Number  enum_struct={}  gain=1  min=-inf  max=inf  precision=''  units=''  help='CAN message value'  group=['Actuators | CAN | ' nam]
  Meas&Ovrd5 : Blocks_lib/Meas&Ovrd  nam=[nam 'NMT_Trg']  name_source=Parameter  view_as=Number  enum_struct={}  gain=1  min=-inf  max=inf  precision=''  units=''  help='CAN message value'  group=['Actuators | CAN | ' nam]
  Meas&Ovrd6 : Blocks_lib/Meas&Ovrd  nam=[nam 'NMT_State']  name_source=Parameter  view_as=Number  enum_struct={}  gain=1  min=-inf  max=inf  precision=''  units=''  help='CAN message value'  group=['Actuators | CAN | ' nam]
  Merge : Merge  Inputs=7
  Off : Subsystem  TreatAsAtomicUnit=on
  Run : Subsystem  TreatAsAtomicUnit=on
  Switch Case : SwitchCase  CaseConditions={[1, 2, 8], 3, 4 ,5 ,6,7,10}  ShowDefaultCase=off
  Terminator : Terminator
  Undefined state : Subsystem  TreatAsAtomicUnit=on
  State : Outport  VectorParamsAs1DForOutWhenUnconnected=off
  wires:
  Undefined state/1(Cmd) -> Merge/1
  Switch Case/1 -> Undefined state/Action
  Bus Creator1/1 -> State/1
  Merge/1 -> Bus Selector1/1
  Bus Selector1/1 -> Inverter Error Reset/2(StateCmd)  "<VCU1StateCmd [bool]>"
  Meas&Ovrd/1 -> Bus Creator1/1  "VCUStateCMD"
  Bus Selector1/2 -> Terminator/1  "<TrqCmd [Nm]>"
  Meas&Ovrd1/1 -> Bus Creator1/2  "StateTrqCmd"
  Bus Selector1/3 -> Meas&Ovrd2/1  "<SpdCmd [rpm]>"
  Meas&Ovrd2/1 -> Bus Creator1/3  "StateSpdCmd"
  Bus Selector1/4 -> Meas&Ovrd3/1  "<VCU1_2_Transmit [bool]>"
  Meas&Ovrd3/1 -> Bus Creator1/4  "VCU12Xmit"
  NMT_Step/1 -> Switch Case/1
  Switch Case/2 -> Init State/Action
  Switch Case/3 -> Off/Action
  Switch Case/4 -> Run/Action
  Switch Case/5 -> Error/Action
  Switch Case/6 -> Error1/Action
  Switch Case/7 -> Error2/Action
  Init State/1(Cmd) -> Merge/2
  Off/1(Cmd) -> Merge/3
  Run/1(Cmd1) -> Merge/4
  Error/1(Cmd) -> Merge/5
  Error1/1(Cmd) -> Merge/6
  Error2/1(Cmd) -> Merge/7
  Bus Selector1/5 -> Meas&Ovrd4/1  "<NMT_Xmit [bool]>"
  Bus Selector1/6 -> Meas&Ovrd5/1  "<NMT_Target_Node>"
  Bus Selector1/7 -> Meas&Ovrd6/1  "<NMT_StateDmd>"
  Meas&Ovrd4/1 -> Bus Creator1/5  "NMTXmit"
  Meas&Ovrd5/1 -> Bus Creator1/6  "NMT_Trg"
  Meas&Ovrd6/1 -> Bus Creator1/7  "NMT_State"
  Data/1 -> Bus Selector/1, Inverter Error Reset/1(Data), Run/1(Input)
  Inverter Error Reset/1(InverterStateCmd) -> Meas&Ovrd/1
  Bus Selector/1 -> Meas&Ovrd1/1  "<DrvMtrTrqReq [Nm]>"

== system VCMGCM1962020b_v2/Fgnd/Actuators/CAN/Drive Inverter/State Transition Command1 ==
  note: TBC: THis needs to be updated per the Saietta interface
      | NOte: WE will use the simple Autostart feature of the drive inverter.
      | THis enables starting without the NMT message handshake
      |
      | Process:
      | Wake all modules
      | Close battery contactors
      | Reset inverter faults
      | Send VCU1/VCU2 Messages
      | Enable inverter in Torque mode.
  NMT_State : Inport
  Data : Inport  Port=2
  Bus Creator1 : BusCreator  Inputs=4
  Bus Selector1 : BusSelector  OutputSignals=AppCtrlCode [bool],TrqCmd [Nm],SpdCmd [rpm],VCU1_2_Transmit [bool]
  Error : Subsystem  TreatAsAtomicUnit=on
  Header : Blocks_lib/Header  width=Portrait  addtext=''
  Init State : Subsystem  TreatAsAtomicUnit=on
  Meas&Ovrd : Blocks_lib/Meas&Ovrd  nam=[nam 'AppStateCmd']  name_source=Parameter  view_as=Number  enum_struct={}  gain=1  min=-inf  max=inf  precision=''  units=''  help='CAN message value'  group=['Actuators | CAN | ' nam]
  Meas&Ovrd1 : Blocks_lib/Meas&Ovrd  nam=[nam 'SateTrqCmd']  name_source=Parameter  view_as=Number  enum_struct={}  gain=1  min=-inf  max=inf  precision=''  units=''  help='CAN message value'  group=['Actuators | CAN | ' nam]
  Meas&Ovrd2 : Blocks_lib/Meas&Ovrd  nam=[nam 'StateSpdCmd']  name_source=Parameter  view_as=Number  enum_struct={}  gain=1  min=-inf  max=inf  precision=''  units=''  help='CAN message value'  group=['Actuators | CAN | ' nam]
  Meas&Ovrd3 : Blocks_lib/Meas&Ovrd  nam=[nam 'VCU12Xmit']  name_source=Parameter  view_as=Number  enum_struct={}  gain=1  min=-inf  max=inf  precision=''  units=''  help='CAN message value'  group=['Actuators | CAN | ' nam]
  Merge : Merge  Inputs=5
  Off : Subsystem  TreatAsAtomicUnit=on
  Run : Subsystem  TreatAsAtomicUnit=on
  Switch Case : SwitchCase  CaseConditions={[-3,-2], -1, 0 ,1 ,2}  ShowDefaultCase=off
  Undefined state : Subsystem  TreatAsAtomicUnit=on
  State : Outport  VectorParamsAs1DForOutWhenUnconnected=off
  wires:
  Switch Case/4 -> Run/Action
  Switch Case/3 -> Off/Action
  Switch Case/2 -> Init State/Action
  Undefined state/1(Cmd) -> Merge/1
  Off/1(Cmd) -> Merge/3
  Run/1(Cmd) -> Merge/4
  Init State/1(Cmd) -> Merge/2
  Switch Case/1 -> Undefined state/Action
  Bus Creator1/1 -> State/1
  Merge/1 -> Bus Selector1/1
  Data/1 -> Run/1(Input), Off/1(Input)
  Bus Selector1/1 -> Meas&Ovrd/1  "<AppCtrlCode [bool]>"
  Meas&Ovrd/1 -> Bus Creator1/1  "AppStateCmd"
  Switch Case/5 -> Error/Action
  Error/1(Cmd) -> Merge/5
  Bus Selector1/2 -> Meas&Ovrd1/1  "<TrqCmd [Nm]>"
  Meas&Ovrd1/1 -> Bus Creator1/2  "StateTrqCmd"
  Bus Selector1/3 -> Meas&Ovrd2/1  "<SpdCmd [rpm]>"
  Meas&Ovrd2/1 -> Bus Creator1/3  "StateSpdCmd"
  Bus Selector1/4 -> Meas&Ovrd3/1  "<VCU1_2_Transmit [bool]>"
  Meas&Ovrd3/1 -> Bus Creator1/4  "VCU12Xmit"
  NMT_State/1 -> Switch Case/1

== system VCMGCM1962020b_v2/Fgnd/Actuators/CAN/Other/A//C Compressor ==
  Data : Inport
  Ground : Ground
  Header : Blocks_lib/Header  width=Portrait  addtext=''
  MsgName : Subsystem  Commented=on
      mask help:
      | Example of how to set up a CAN message transmit.
      | 1. Copy this block into the main model.
      | 2. Disable/break library link.
      | 3. Underneath, set up CAN Tx Message block.
      | 4. For each field, connect a CANTxField block from the CAN block to the bus creator; adjust parameters as necessary.
      mask init:
      | [msgnam, msgbus] = CANBlockInit('Tx');
      mask Display: disp(['CAN Tx: Message\n' msgnam '\n' msgbus]);
  Act : Outport  VectorParamsAs1DForOutWhenUnconnected=off
  wires:
  Ground/1 -> Act/1  "ACC"
  Data/1 -> MsgName/1(Data)

== system VCMGCM1962020b_v2/Fgnd/Actuators/CAN/Other/Cooling Pump 1 ==
  Data : Inport
  Ground : Ground
  Header : Blocks_lib/Header  width=Portrait  addtext=''
  MsgName : Subsystem
      mask help:
      | Example of how to set up a CAN message transmit.
      | 1. Copy this block into the main model.
      | 2. Disable/break library link.
      | 3. Underneath, set up CAN Tx Message block.
      | 4. For each field, connect a CANTxField block from the CAN block to the bus creator; adjust parameters as necessary.
      mask init:
      | [msgnam, msgbus] = CANBlockInit('Tx');
      mask Display: disp(['CAN Tx: Message\n' msgnam '\n' msgbus]);
  Act : Outport  VectorParamsAs1DForOutWhenUnconnected=off
  wires:
  Data/1 -> MsgName/1(Data)
  Ground/1 -> Act/1  "CoolPump1"

== system VCMGCM1962020b_v2/Fgnd/Actuators/CAN/Other/Cooling Pump 2 ==
  Data : Inport
  Ground : Ground
  Header : Blocks_lib/Header  width=Portrait  addtext=''
  MsgName : Subsystem
      mask help:
      | Example of how to set up a CAN message transmit.
      | 1. Copy this block into the main model.
      | 2. Disable/break library link.
      | 3. Underneath, set up CAN Tx Message block.
      | 4. For each field, connect a CANTxField block from the CAN block to the bus creator; adjust parameters as necessary.
      mask init:
      | [msgnam, msgbus] = CANBlockInit('Tx');
      mask Display: disp(['CAN Tx: Message\n' msgnam '\n' msgbus]);
  Act : Outport  VectorParamsAs1DForOutWhenUnconnected=off
  wires:
  Ground/1 -> Act/1  "CoolPump2"
  Data/1 -> MsgName/1(Data)

== system VCMGCM1962020b_v2/Fgnd/Actuators/CAN/Other/Heater ==
  Data : Inport
  Ground : Ground
  Header : Blocks_lib/Header  width=Portrait  addtext=''
  MsgName : Subsystem
      mask help:
      | Example of how to set up a CAN message transmit.
      | 1. Copy this block into the main model.
      | 2. Disable/break library link.
      | 3. Underneath, set up CAN Tx Message block.
      | 4. For each field, connect a CANTxField block from the CAN block to the bus creator; adjust parameters as necessary.
      mask init:
      | [msgnam, msgbus] = CANBlockInit('Tx');
      mask Display: disp(['CAN Tx: Message\n' msgnam '\n' msgbus]);
  Act : Outport  VectorParamsAs1DForOutWhenUnconnected=off
  wires:
  Data/1 -> MsgName/1(Data)
  Ground/1 -> Act/1  "Heater"
